simulink model "hexacopter"  (R2023b)
settings: Solver=ode3  StartTime=0.0  StopTime=inf  FixedStep=0.005  RelTol=1e-3
values from neighbouring files (symbols this model uses):
  A = [zeros(4),eye(4) ... (first row only)    [hexacopter_params.m]
  B = [0 0 0 0 ... (first row only)    [hexa.m]    (also in hexacopter_params.m = [zeros(4))
  body_params = [L,b,d,m,Ix,Iy,Iz,J_T]    [hexacopter_params.m]
  C = eye(8)    [hexacopter_params.m]
  g = 9.82    [hexacopter_params.m]
  K = place(A', C', desired_poles)'    [hexacopter_params.m]
  m = 2.5    [hexacopter_params.m]
  Simulation_params = [g,K_phi,K_theta,K_psi,K_x,K_y,K_z]    [hexacopter_params.m]
  T = [1, 1, 1, 1, 1, 1 ... (first row only)    [hexacopter_params.m]
  T_inv = pinv(T)    [hexacopter_params.m]
libraries: slpidlib x5, aerolibutil x2, vrlib x2
(part 1 of 2)
settings Model: Creator=alexe  LastModifiedBy=Therkelsen

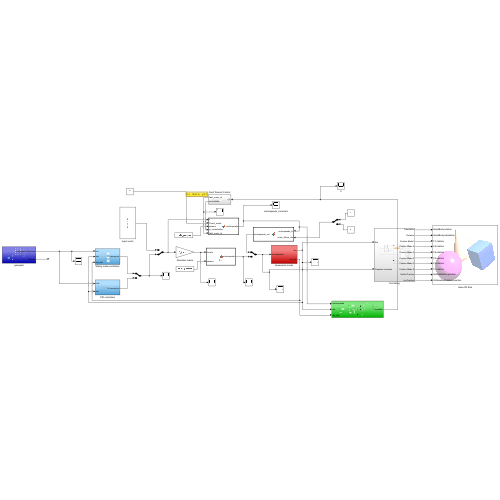
[thumbnail: Simulink's stored preview of the top-level diagram]
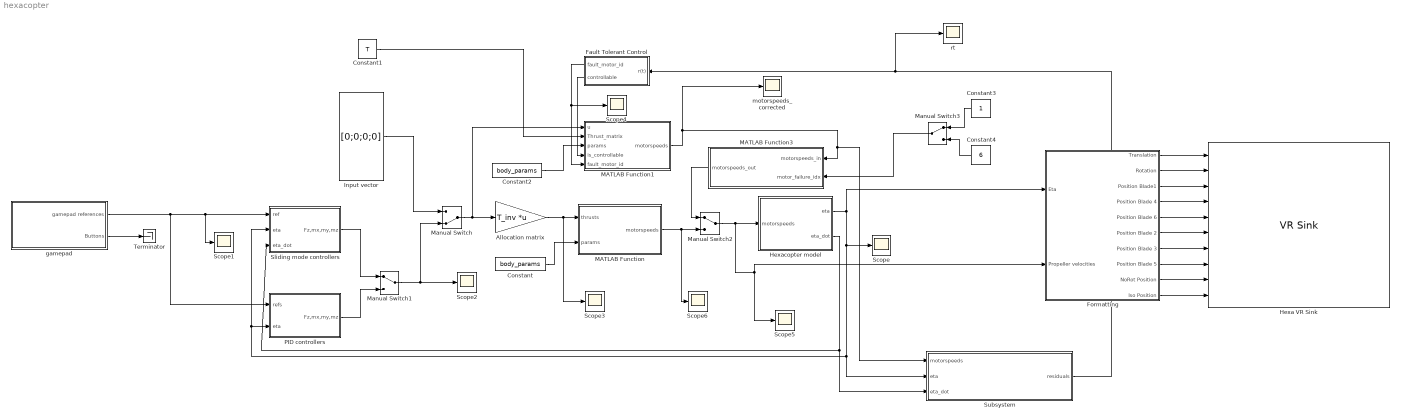
== system hexacopter ==
  Allocation matrix : Gain  Gain=T_inv  Multiplication=Matrix(K*u)
  Constant : Constant  Value=body_params
  Constant1 : Constant  Value=T
  Constant2 : Constant  Value=body_params
  Constant3 : Constant
  Constant4 : Constant  Value=6
  Fault Tolerant Control : Subsystem
  Formatting : Subsystem
  Hexa VR Sink : vrlib/VR Sink  InstantiateOnLoad=on  SampleTime=12*0.005  ViewEnable=on  RemoteChange=off  RemoteView=off  FieldsWritten=QuadBody.rotation.4.1.1.double#QuadBody.translation.3.1.1.double#F1.rotation.4.1.1.double#F4.rotation.4.1.1.double#F6.rotation.4.1.1.double#F2.rotation.4.1.1.double#F3.rotation.4.1.1.double#F5.rotation.4.1.1.double#IsoNoRotation.position.3.1.1.double#OnQuadNoRotation.position.3.1.1.double  WorldFileName=Hexacopter_VR.wrl  AutoView=on  VideoDimensions=[]  AllowVariableSize=off
  Hexacopter model : Subsystem
  Input vector : Constant  Value=[0;0;0;0]  VectorParams1D=off
  MATLAB Function : MATLAB Function  TreatAsAtomicUnit=on
  MATLAB Function1 : MATLAB Function  TreatAsAtomicUnit=on
  MATLAB Function3 : MATLAB Function  TreatAsAtomicUnit=on
  Manual Switch : ManualSwitch  CurrentSetting=0
  Manual Switch1 : ManualSwitch
  Manual Switch2 : ManualSwitch
  Manual Switch3 : ManualSwitch
  PID controllers : Subsystem
  Scope{,1..6} (7 alike) : Scope
  Sliding mode controllers : Subsystem
  Subsystem : Subsystem
  Terminator : Terminator
  gamepad : Subsystem
  motorspeeds_corrected : Scope
  rt : Scope
  wires:
  Allocation matrix/1 -> Scope3/1, MATLAB Function/1(thrusts)
  Manual Switch/1 -> MATLAB Function1/1(u), Allocation matrix/1
  Input vector/1 -> Manual Switch/1
  PID controllers/1(Fz,mx,my,mz) -> Manual Switch1/2
  Manual Switch1/1 -> Manual Switch/2, Scope2/1
  Sliding mode controllers/1(Fz,mx,my,mz) -> Manual Switch1/1
  Constant/1 -> MATLAB Function/2(params)
  Hexacopter model/2(eta_dot) -> Sliding mode controllers/3(eta_dot), Subsystem/3(eta_dot)
  MATLAB Function/1(motorspeeds) -> Scope6/1, Manual Switch2/2
  MATLAB Function1/1(motorspeeds) -> motorspeeds_corrected/1, Subsystem/1(motorspeeds), MATLAB Function3/1(motorspeeds_in)
  Constant2/1 -> MATLAB Function1/3(params)
  gamepad/1(gamepad references) -> PID controllers/1(refs), Scope1/1, Sliding mode controllers/1(ref)
  MATLAB Function3/1(motorspeeds_out) -> Manual Switch2/1
  Subsystem/1(residuals) -> rt/1, Fault Tolerant Control/1(r(t))
  Constant1/1 -> MATLAB Function1/2(Thrust_matrix)
  Fault Tolerant Control/2(controllable) -> MATLAB Function1/4(is_controllable)
  Constant4/1 -> Manual Switch3/2
  Manual Switch3/1 -> MATLAB Function3/2(motor_failure_idx)
  gamepad/2(Buttons) -> Terminator/1
  Fault Tolerant Control/1(fault_motor_id) -> Scope4/1, MATLAB Function1/5(fault_motor_id)
  Constant3/1 -> Manual Switch3/1
  Formatting/7(Position Blade 3) -> Hexa VR Sink/7
  Formatting/6(Position Blade 2) -> Hexa VR Sink/6
  Formatting/9(NoRot Position) -> Hexa VR Sink/9
  Formatting/10(Iso Position) -> Hexa VR Sink/10
  Formatting/3(Position Blade1) -> Hexa VR Sink/3
  Formatting/1(Translation) -> Hexa VR Sink/1
  Formatting/8(Position Blade 5) -> Hexa VR Sink/8
  Formatting/4(Position Blade 4) -> Hexa VR Sink/4
  Manual Switch2/1 -> Scope5/1, Formatting/2(Propeller velocities), Hexacopter model/1(motorspeeds)
  Formatting/5(Position Blade 6) -> Hexa VR Sink/5
  Hexacopter model/1(eta) -> Formatting/1(Eta), PID controllers/2(eta), Sliding mode controllers/2(eta), Subsystem/2(eta), Scope/1
  Formatting/2(Rotation) -> Hexa VR Sink/2

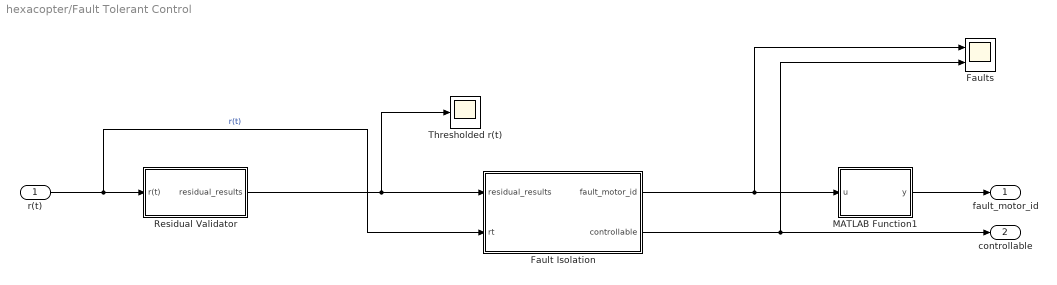
== system hexacopter/Fault Tolerant Control ==
  r(t) : Inport
  Fault Isolation : Subsystem
  Faults : Scope  NumInputPorts=2
  MATLAB Function1 : MATLAB Function  TreatAsAtomicUnit=on
  Residual Validator : Subsystem
  Thresholded r(t) : Scope
  fault_motor_id : Outport
  controllable : Outport  Port=2
  wires:
  Fault Isolation/1(fault_motor_id) -> MATLAB Function1/1(u), Faults/1
  Fault Isolation/2(controllable) -> Faults/2, controllable/1
  r(t)/1 -> Fault Isolation/2(rt), Residual Validator/1(r(t))  "r(t)"
  Residual Validator/1(residual_results) -> Fault Isolation/1(residual_results), Thresholded r(t)/1
  MATLAB Function1/1(y) -> fault_motor_id/1

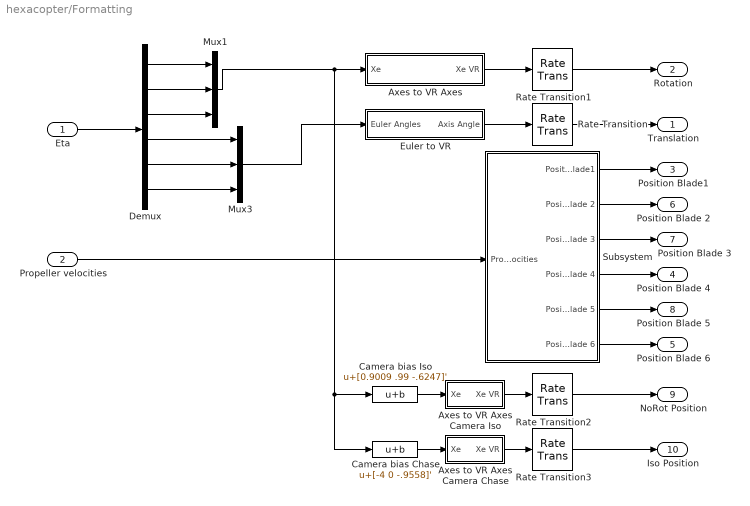
== system hexacopter/Formatting ==
  Eta : Inport
  Propeller velocities : Inport  Port=2
  Axes to VR Axes : Subsystem
  Axes to VR Axes Camera Chase : Subsystem
  Axes to VR Axes Camera Iso : Subsystem
  Camera bias Chase : Bias  Bias=[-4 0 -.9558]'  SaturateOnIntegerOverflow=off
  Camera bias Iso : Bias  Bias=[0.9009 .99 -.6247]'  SaturateOnIntegerOverflow=off
  Demux : Demux  Outputs=6
  Euler to VR : Subsystem
  Mux1 : Mux  Inputs=3
  Mux3 : Mux  Inputs=3
  Rate Transition{,1..3} (4 alike) : RateTransition
  Subsystem : Subsystem
  Translation : Outport
  Rotation : Outport  Port=2
  Position Blade1 : Outport  Port=3
  Position Blade 4 : Outport  Port=4
  Position Blade 6 : Outport  Port=5
  Position Blade 2 : Outport  Port=6
  Position Blade 3 : Outport  Port=7
  Position Blade 5 : Outport  Port=8
  NoRot Position : Outport  Port=9
  Iso Position : Outport  Port=10
  wires:
  Rate Transition2/1 -> NoRot Position/1
  Propeller velocities/1 -> Subsystem/1(Propeller velocities)
  Subsystem/3(Position Blade 3) -> Position Blade 3/1
  Subsystem/1(Position Blade1) -> Position Blade1/1
  Mux3/1 -> Euler to VR/1(Euler Angles)
  Camera bias Chase/1 -> Axes to VR Axes Camera Chase/1(Xe)
  Axes to VR Axes Camera Chase/1(Xe VR) -> Rate Transition3/1
  Subsystem/2(Position Blade 2) -> Position Blade 2/1
  Axes to VR Axes Camera Iso/1(Xe VR) -> Rate Transition2/1
  Euler to VR/1(Axis Angle) -> Rate Transition/1
  Axes to VR Axes/1(Xe VR) -> Rate Transition1/1
  Rate Transition1/1 -> Rotation/1
  Camera bias Iso/1 -> Axes to VR Axes Camera Iso/1(Xe)
  Mux1/1 -> Camera bias Chase/1, Camera bias Iso/1, Axes to VR Axes/1(Xe)
  Rate Transition3/1 -> Iso Position/1
  Rate Transition/1 -> Translation/1
  Subsystem/4(Position Blade 4) -> Position Blade 4/1
  Demux/2 -> Mux1/2
  Demux/5 -> Mux3/2
  Demux/3 -> Mux1/3
  Eta/1 -> Demux/1
  Demux/1 -> Mux1/1
  Demux/4 -> Mux3/1
  Demux/6 -> Mux3/3
  Subsystem/6(Position Blade 6) -> Position Blade 6/1
  Subsystem/5(Position Blade 5) -> Position Blade 5/1

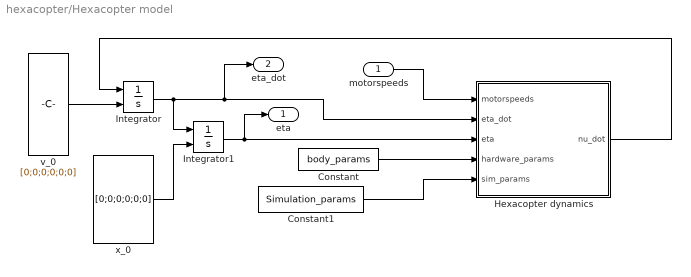
== system hexacopter/Hexacopter model ==
  motorspeeds : Inport
  Constant : Constant  Value=body_params
  Constant1 : Constant  Value=Simulation_params
  Hexacopter dynamics : MATLAB Function  TreatAsAtomicUnit=on
  Integrator : Integrator  InitialConditionSource=external
  Integrator1 : Integrator  InitialConditionSource=external
  v_0 : Constant  Value=[0;0;0;0;0;0]  VectorParams1D=off
  x_0 : Constant  Value=[0;0;0;0;0;0]  VectorParams1D=off
  eta : Outport
  eta_dot : Outport  Port=2
  wires:
  motorspeeds/1 -> Hexacopter dynamics/1(motorspeeds)
  Integrator/1 -> Integrator1/1, Hexacopter dynamics/2(eta_dot), eta_dot/1
  Integrator1/1 -> Hexacopter dynamics/3(eta), eta/1
  Hexacopter dynamics/1(nu_dot) -> Integrator/1
  v_0/1 -> Integrator/2
  Constant1/1 -> Hexacopter dynamics/5(sim_params)
  x_0/1 -> Integrator1/2
  Constant/1 -> Hexacopter dynamics/4(hardware_params)

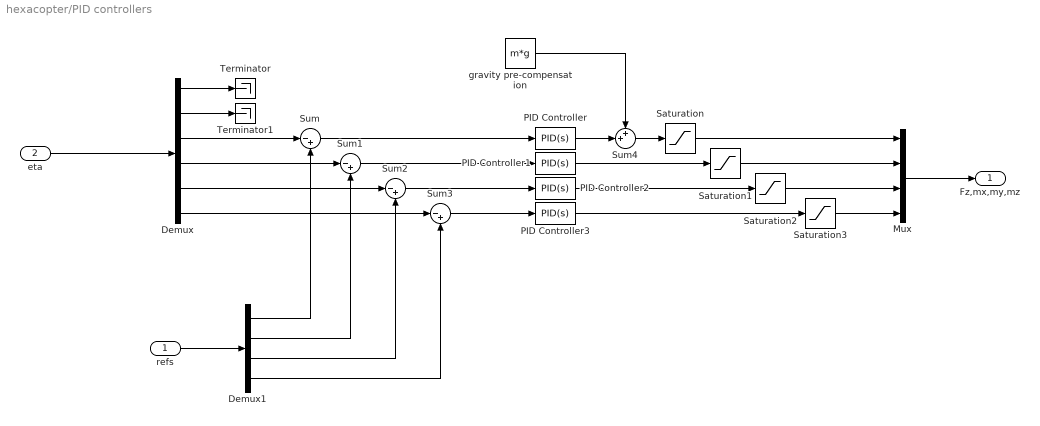
== system hexacopter/PID controllers ==
  refs : Inport
  eta : Inport  Port=2
  Demux : Demux  Outputs=6
  Demux1 : Demux
  Mux : Mux
  PID Controller : slpidlib/PID Controller  Controller=PID  Form=Parallel  TimeDomain=Continuous-time  UseExternalTs=off  SampleTime=-1  IntegratorMethod=Forward Euler  FilterMethod=Forward Euler  ControllerParametersSource=internal  P=3  I=1  UseKiTs=off  D=8  N=100  UseFilter=on  TunerSelectOption=Transfer Function Based (PID Tuner App)  InitialConditionSource=internal  InitialConditionForIntegrator=0  InitialConditionForFilter=0  DifferentiatorICPrevScaledInput=0  ExternalReset=none  TrackingMode=off  Kt=1  LimitOutput=off  SatLimitsSource=internal  UpperSaturationLimit=inf  LowerSaturationLimit=-inf  LinearizeAsGain=on  AntiWindupMode=none  Kb=1  LimitIntegrator=off  UpperIntegratorSaturationLimit=inf  LowerIntegratorSaturationLimit=-inf  POutMin=[]  POutMax=[]  IOutMin=[]  IOutMax=[]  DOutMin=[]  DOutMax=[]  NOutMin=[]  NOutMax=[]  SumOutMin=[]  SumOutMax=[]  SaturationOutMin=[]  SaturationOutMax=[]  PParamMin=[]  PParamMax=[]  IParamMin=[]  IParamMax=[]  DParamMin=[]  DParamMax=[]  NParamMin=[]  NParamMax=[]  KbParamMin=[]  KbParamMax=[]  KtParamMin=[]  KtParamMax=[]  KbOutMin=[]  KbOutMax=[]  KtOutMin=[]  KtOutMax=[]  IntegratorOutMin=[]  IntegratorOutMax=[]  FilterOutMin=[]  FilterOutMax=[]  SumI1OutMin=[]  SumI1OutMax=[]  SumI2OutMin=[]  SumI2OutMax=[]  SumI3OutMin=[]  SumI3OutMax=[]  SumI4OutMin=[]  SumI4OutMax=[]  SumDOutMin=[]  SumDOutMax=[]  DifferentiatorOutMin=[]  DifferentiatorOutMax=[]  FilterDiffOutCoefMin=[]  FilterDiffOutCoefMax=[]  ReciprocalOutMin=[]  ReciprocalOutMax=[]  SumDenOutMin=[]  SumDenOutMax=[]  SumNumOutMin=[]  SumNumOutMax=[]  DivideOutMin=[]  DivideOutMax=[]  UdiffTsProdOutMin=[]  UdiffTsProdOutMax=[]  NTsProdOutMin=[]  NTsProdOutMax=[]  UintegralTsProdOutMin=[]  UintegralTsProdOutMax=[]  UngainTsProdOutMin=[]  UngainTsProdOutMax=[]  ClampingZeroOutDataTypeStr=Inherit: Inherit via back propagation  ClampingZeroOutMin=[]  ClampingZeroOutMax=[]  FilterDenConstantOutDataTypeStr=Inherit: Inherit via back propagation  FilterDenConstantOutMin=[]  FilterDenConstantOutMax=[]  PCopyOutDataTypeStr=Inherit: Inherit via back propagation  PCopyOutMin=[]  PCopyOutMax=[]  NCopyOutDataTypeStr=Inherit: Inherit via back propagation  NCopyOutMin=[]  NCopyOutMax=[]  IntegratorContinuousStateAttributes=''  IntegratorStateMustResolveToSignalObject=off  IntegratorRTWStateStorageClass=Auto  FilterContinuousStateAttributes=''  FilterStateMustResolveToSignalObject=off  FilterRTWStateStorageClass=Auto  ParallelPVariant=InternalParameters  IdealPVariant=Disabled  IVariant=InternalParameters  DVariant=InternalParameters  IntegratorVariant=Continuous  SatVariant=Disabled  AWVariant=Passthrough  PCopyVariant=Disabled  TRVariant=Disabled  FdbkBlocksVariant=Forward  IdealPFdbkVariant=Disabled  SatFdbkVariant=Disabled  DerivativeFilterVariant=ContFilter  NVariant=InternalParameters  NCopyVariant=Disabled  FilterICVariant=InternalICsFilter  IntegratorICVariant=InternalICs  ExternalResetVariant=Disabled  TRSumVariant=Passthrough  SumFdbkVariant=Disabled  SumVariant=Sum_PID  TsampFilterVariant=InternalTs  TsampNgainVariant=Passthrough  TsampIntegralVariant=Disabled_SignalSpec  ExternalSaturationOutDataTypeStr=Inherit: Same as second input
  PID Controller1 : slpidlib/PID Controller  Controller=PID  Form=Parallel  TimeDomain=Continuous-time  UseExternalTs=off  SampleTime=-1  IntegratorMethod=Forward Euler  FilterMethod=Forward Euler  ControllerParametersSource=internal  P=1  I=0  UseKiTs=off  D=5  N=100  UseFilter=on  TunerSelectOption=Transfer Function Based (PID Tuner App)  InitialConditionSource=internal  InitialConditionForIntegrator=0  InitialConditionForFilter=0  DifferentiatorICPrevScaledInput=0  ExternalReset=none  TrackingMode=off  Kt=1  LimitOutput=off  SatLimitsSource=internal  UpperSaturationLimit=inf  LowerSaturationLimit=-inf  LinearizeAsGain=on  AntiWindupMode=none  Kb=1  LimitIntegrator=off  UpperIntegratorSaturationLimit=inf  LowerIntegratorSaturationLimit=-inf  POutMin=[]  POutMax=[]  IOutMin=[]  IOutMax=[]  DOutMin=[]  DOutMax=[]  NOutMin=[]  NOutMax=[]  SumOutMin=[]  SumOutMax=[]  SaturationOutMin=[]  SaturationOutMax=[]  PParamMin=[]  PParamMax=[]  IParamMin=[]  IParamMax=[]  DParamMin=[]  DParamMax=[]  NParamMin=[]  NParamMax=[]  KbParamMin=[]  KbParamMax=[]  KtParamMin=[]  KtParamMax=[]  KbOutMin=[]  KbOutMax=[]  KtOutMin=[]  KtOutMax=[]  IntegratorOutMin=[]  IntegratorOutMax=[]  FilterOutMin=[]  FilterOutMax=[]  SumI1OutMin=[]  SumI1OutMax=[]  SumI2OutMin=[]  SumI2OutMax=[]  SumI3OutMin=[]  SumI3OutMax=[]  SumI4OutMin=[]  SumI4OutMax=[]  SumDOutMin=[]  SumDOutMax=[]  DifferentiatorOutMin=[]  DifferentiatorOutMax=[]  FilterDiffOutCoefMin=[]  FilterDiffOutCoefMax=[]  ReciprocalOutMin=[]  ReciprocalOutMax=[]  SumDenOutMin=[]  SumDenOutMax=[]  SumNumOutMin=[]  SumNumOutMax=[]  DivideOutMin=[]  DivideOutMax=[]  UdiffTsProdOutMin=[]  UdiffTsProdOutMax=[]  NTsProdOutMin=[]  NTsProdOutMax=[]  UintegralTsProdOutMin=[]  UintegralTsProdOutMax=[]  UngainTsProdOutMin=[]  UngainTsProdOutMax=[]  ClampingZeroOutDataTypeStr=Inherit: Inherit via back propagation  ClampingZeroOutMin=[]  ClampingZeroOutMax=[]  FilterDenConstantOutDataTypeStr=Inherit: Inherit via back propagation  FilterDenConstantOutMin=[]  FilterDenConstantOutMax=[]  PCopyOutDataTypeStr=Inherit: Inherit via back propagation  PCopyOutMin=[]  PCopyOutMax=[]  NCopyOutDataTypeStr=Inherit: Inherit via back propagation  NCopyOutMin=[]  NCopyOutMax=[]  IntegratorContinuousStateAttributes=''  IntegratorStateMustResolveToSignalObject=off  IntegratorRTWStateStorageClass=Auto  FilterContinuousStateAttributes=''  FilterStateMustResolveToSignalObject=off  FilterRTWStateStorageClass=Auto  ParallelPVariant=InternalParameters  IdealPVariant=Disabled  IVariant=InternalParameters  DVariant=InternalParameters  IntegratorVariant=Continuous  SatVariant=Disabled  AWVariant=Passthrough  PCopyVariant=Disabled  TRVariant=Disabled  FdbkBlocksVariant=Forward  IdealPFdbkVariant=Disabled  SatFdbkVariant=Disabled  DerivativeFilterVariant=ContFilter  NVariant=InternalParameters  NCopyVariant=Disabled  FilterICVariant=InternalICsFilter  IntegratorICVariant=InternalICs  ExternalResetVariant=Disabled  TRSumVariant=Passthrough  SumFdbkVariant=Disabled  SumVariant=Sum_PID  TsampFilterVariant=InternalTs  TsampNgainVariant=Passthrough  TsampIntegralVariant=Disabled_SignalSpec  ExternalSaturationOutDataTypeStr=Inherit: Same as second input
  PID Controller2 : slpidlib/PID Controller  Controller=PID  Form=Parallel  TimeDomain=Continuous-time  UseExternalTs=off  SampleTime=-1  IntegratorMethod=Forward Euler  FilterMethod=Forward Euler  ControllerParametersSource=internal  P=1  I=0  UseKiTs=off  D=5  N=100  UseFilter=on  TunerSelectOption=Transfer Function Based (PID Tuner App)  InitialConditionSource=internal  InitialConditionForIntegrator=0  InitialConditionForFilter=0  DifferentiatorICPrevScaledInput=0  ExternalReset=none  TrackingMode=off  Kt=1  LimitOutput=off  SatLimitsSource=internal  UpperSaturationLimit=inf  LowerSaturationLimit=-inf  LinearizeAsGain=on  AntiWindupMode=none  Kb=1  LimitIntegrator=off  UpperIntegratorSaturationLimit=inf  LowerIntegratorSaturationLimit=-inf  POutMin=[]  POutMax=[]  IOutMin=[]  IOutMax=[]  DOutMin=[]  DOutMax=[]  NOutMin=[]  NOutMax=[]  SumOutMin=[]  SumOutMax=[]  SaturationOutMin=[]  SaturationOutMax=[]  PParamMin=[]  PParamMax=[]  IParamMin=[]  IParamMax=[]  DParamMin=[]  DParamMax=[]  NParamMin=[]  NParamMax=[]  KbParamMin=[]  KbParamMax=[]  KtParamMin=[]  KtParamMax=[]  KbOutMin=[]  KbOutMax=[]  KtOutMin=[]  KtOutMax=[]  IntegratorOutMin=[]  IntegratorOutMax=[]  FilterOutMin=[]  FilterOutMax=[]  SumI1OutMin=[]  SumI1OutMax=[]  SumI2OutMin=[]  SumI2OutMax=[]  SumI3OutMin=[]  SumI3OutMax=[]  SumI4OutMin=[]  SumI4OutMax=[]  SumDOutMin=[]  SumDOutMax=[]  DifferentiatorOutMin=[]  DifferentiatorOutMax=[]  FilterDiffOutCoefMin=[]  FilterDiffOutCoefMax=[]  ReciprocalOutMin=[]  ReciprocalOutMax=[]  SumDenOutMin=[]  SumDenOutMax=[]  SumNumOutMin=[]  SumNumOutMax=[]  DivideOutMin=[]  DivideOutMax=[]  UdiffTsProdOutMin=[]  UdiffTsProdOutMax=[]  NTsProdOutMin=[]  NTsProdOutMax=[]  UintegralTsProdOutMin=[]  UintegralTsProdOutMax=[]  UngainTsProdOutMin=[]  UngainTsProdOutMax=[]  ClampingZeroOutDataTypeStr=Inherit: Inherit via back propagation  ClampingZeroOutMin=[]  ClampingZeroOutMax=[]  FilterDenConstantOutDataTypeStr=Inherit: Inherit via back propagation  FilterDenConstantOutMin=[]  FilterDenConstantOutMax=[]  PCopyOutDataTypeStr=Inherit: Inherit via back propagation  PCopyOutMin=[]  PCopyOutMax=[]  NCopyOutDataTypeStr=Inherit: Inherit via back propagation  NCopyOutMin=[]  NCopyOutMax=[]  IntegratorContinuousStateAttributes=''  IntegratorStateMustResolveToSignalObject=off  IntegratorRTWStateStorageClass=Auto  FilterContinuousStateAttributes=''  FilterStateMustResolveToSignalObject=off  FilterRTWStateStorageClass=Auto  ParallelPVariant=InternalParameters  IdealPVariant=Disabled  IVariant=InternalParameters  DVariant=InternalParameters  IntegratorVariant=Continuous  SatVariant=Disabled  AWVariant=Passthrough  PCopyVariant=Disabled  TRVariant=Disabled  FdbkBlocksVariant=Forward  IdealPFdbkVariant=Disabled  SatFdbkVariant=Disabled  DerivativeFilterVariant=ContFilter  NVariant=InternalParameters  NCopyVariant=Disabled  FilterICVariant=InternalICsFilter  IntegratorICVariant=InternalICs  ExternalResetVariant=Disabled  TRSumVariant=Passthrough  SumFdbkVariant=Disabled  SumVariant=Sum_PID  TsampFilterVariant=InternalTs  TsampNgainVariant=Passthrough  TsampIntegralVariant=Disabled_SignalSpec  ExternalSaturationOutDataTypeStr=Inherit: Same as second input
  PID Controller3 : slpidlib/PID Controller  Controller=PID  Form=Parallel  TimeDomain=Continuous-time  UseExternalTs=off  SampleTime=-1  IntegratorMethod=Forward Euler  FilterMethod=Forward Euler  ControllerParametersSource=internal  P=1  I=0  UseKiTs=off  D=3  N=100  UseFilter=on  TunerSelectOption=Transfer Function Based (PID Tuner App)  InitialConditionSource=internal  InitialConditionForIntegrator=0  InitialConditionForFilter=0  DifferentiatorICPrevScaledInput=0  ExternalReset=none  TrackingMode=off  Kt=1  LimitOutput=off  SatLimitsSource=internal  UpperSaturationLimit=inf  LowerSaturationLimit=-inf  LinearizeAsGain=on  AntiWindupMode=none  Kb=1  LimitIntegrator=off  UpperIntegratorSaturationLimit=inf  LowerIntegratorSaturationLimit=-inf  POutMin=[]  POutMax=[]  IOutMin=[]  IOutMax=[]  DOutMin=[]  DOutMax=[]  NOutMin=[]  NOutMax=[]  SumOutMin=[]  SumOutMax=[]  SaturationOutMin=[]  SaturationOutMax=[]  PParamMin=[]  PParamMax=[]  IParamMin=[]  IParamMax=[]  DParamMin=[]  DParamMax=[]  NParamMin=[]  NParamMax=[]  KbParamMin=[]  KbParamMax=[]  KtParamMin=[]  KtParamMax=[]  KbOutMin=[]  KbOutMax=[]  KtOutMin=[]  KtOutMax=[]  IntegratorOutMin=[]  IntegratorOutMax=[]  FilterOutMin=[]  FilterOutMax=[]  SumI1OutMin=[]  SumI1OutMax=[]  SumI2OutMin=[]  SumI2OutMax=[]  SumI3OutMin=[]  SumI3OutMax=[]  SumI4OutMin=[]  SumI4OutMax=[]  SumDOutMin=[]  SumDOutMax=[]  DifferentiatorOutMin=[]  DifferentiatorOutMax=[]  FilterDiffOutCoefMin=[]  FilterDiffOutCoefMax=[]  ReciprocalOutMin=[]  ReciprocalOutMax=[]  SumDenOutMin=[]  SumDenOutMax=[]  SumNumOutMin=[]  SumNumOutMax=[]  DivideOutMin=[]  DivideOutMax=[]  UdiffTsProdOutMin=[]  UdiffTsProdOutMax=[]  NTsProdOutMin=[]  NTsProdOutMax=[]  UintegralTsProdOutMin=[]  UintegralTsProdOutMax=[]  UngainTsProdOutMin=[]  UngainTsProdOutMax=[]  ClampingZeroOutDataTypeStr=Inherit: Inherit via back propagation  ClampingZeroOutMin=[]  ClampingZeroOutMax=[]  FilterDenConstantOutDataTypeStr=Inherit: Inherit via back propagation  FilterDenConstantOutMin=[]  FilterDenConstantOutMax=[]  PCopyOutDataTypeStr=Inherit: Inherit via back propagation  PCopyOutMin=[]  PCopyOutMax=[]  NCopyOutDataTypeStr=Inherit: Inherit via back propagation  NCopyOutMin=[]  NCopyOutMax=[]  IntegratorContinuousStateAttributes=''  IntegratorStateMustResolveToSignalObject=off  IntegratorRTWStateStorageClass=Auto  FilterContinuousStateAttributes=''  FilterStateMustResolveToSignalObject=off  FilterRTWStateStorageClass=Auto  ParallelPVariant=InternalParameters  IdealPVariant=Disabled  IVariant=InternalParameters  DVariant=InternalParameters  IntegratorVariant=Continuous  SatVariant=Disabled  AWVariant=Passthrough  PCopyVariant=Disabled  TRVariant=Disabled  FdbkBlocksVariant=Forward  IdealPFdbkVariant=Disabled  SatFdbkVariant=Disabled  DerivativeFilterVariant=ContFilter  NVariant=InternalParameters  NCopyVariant=Disabled  FilterICVariant=InternalICsFilter  IntegratorICVariant=InternalICs  ExternalResetVariant=Disabled  TRSumVariant=Passthrough  SumFdbkVariant=Disabled  SumVariant=Sum_PID  TsampFilterVariant=InternalTs  TsampNgainVariant=Passthrough  TsampIntegralVariant=Disabled_SignalSpec  ExternalSaturationOutDataTypeStr=Inherit: Same as second input
  Saturation : Saturate  UpperLimit=100  LowerLimit=-100
  Saturation1 : Saturate  UpperLimit=5  LowerLimit=-5
  Saturation2 : Saturate  UpperLimit=5  LowerLimit=-5
  Saturation3 : Saturate  UpperLimit=5  LowerLimit=-5
  Sum{,1..3} (4 alike) : Sum  Inputs=|-+
  Sum4 : Sum  Inputs=++|
  Terminator : Terminator
  Terminator1 : Terminator
  gravity pre-compensation : Constant  Value=m*g
  Fz,mx,my,mz : Outport
  wires:
  eta/1 -> Demux/1
  refs/1 -> Demux1/1
  Demux/1 -> Terminator/1
  Demux/2 -> Terminator1/1
  Demux/3 -> Sum/1
  Demux1/1 -> Sum/2
  Demux/4 -> Sum1/1
  Demux1/2 -> Sum1/2
  Demux/5 -> Sum2/1
  Demux1/3 -> Sum2/2
  Demux/6 -> Sum3/1
  Demux1/4 -> Sum3/2
  Sum/1 -> PID Controller/1
  Sum1/1 -> PID Controller1/1
  Sum2/1 -> PID Controller2/1
  Sum3/1 -> PID Controller3/1
  PID Controller3/1 -> Saturation3/1
  PID Controller2/1 -> Saturation2/1
  PID Controller1/1 -> Saturation1/1
  Mux/1 -> Fz,mx,my,mz/1
  Sum4/1 -> Saturation/1
  PID Controller/1 -> Sum4/2
  gravity pre-compensation/1 -> Sum4/1
  Saturation/1 -> Mux/1
  Saturation1/1 -> Mux/2
  Saturation2/1 -> Mux/3
  Saturation3/1 -> Mux/4

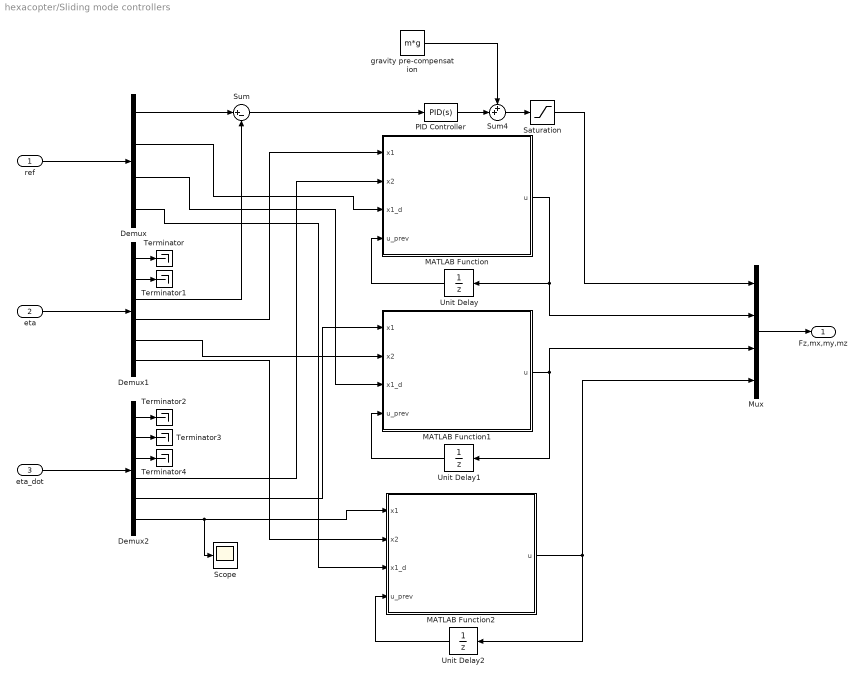
== system hexacopter/Sliding mode controllers ==
  ref : Inport
  eta : Inport  Port=2
  eta_dot : Inport  Port=3
  Demux : Demux
  Demux1 : Demux  Outputs=6
  Demux2 : Demux  Outputs=6
  MATLAB Function : MATLAB Function  TreatAsAtomicUnit=on
  MATLAB Function1 : MATLAB Function  TreatAsAtomicUnit=on
  MATLAB Function2 : MATLAB Function  TreatAsAtomicUnit=on
  Mux : Mux
  PID Controller : slpidlib/PID Controller  Controller=PID  Form=Parallel  TimeDomain=Continuous-time  UseExternalTs=off  SampleTime=-1  IntegratorMethod=Forward Euler  FilterMethod=Forward Euler  ControllerParametersSource=internal  P=3  I=1  UseKiTs=off  D=8  N=100  UseFilter=on  TunerSelectOption=Transfer Function Based (PID Tuner App)  InitialConditionSource=internal  InitialConditionForIntegrator=0  InitialConditionForFilter=0  DifferentiatorICPrevScaledInput=0  ExternalReset=none  TrackingMode=off  Kt=1  LimitOutput=off  SatLimitsSource=internal  UpperSaturationLimit=inf  LowerSaturationLimit=-inf  LinearizeAsGain=on  AntiWindupMode=none  Kb=1  LimitIntegrator=off  UpperIntegratorSaturationLimit=inf  LowerIntegratorSaturationLimit=-inf  POutMin=[]  POutMax=[]  IOutMin=[]  IOutMax=[]  DOutMin=[]  DOutMax=[]  NOutMin=[]  NOutMax=[]  SumOutMin=[]  SumOutMax=[]  SaturationOutMin=[]  SaturationOutMax=[]  PParamMin=[]  PParamMax=[]  IParamMin=[]  IParamMax=[]  DParamMin=[]  DParamMax=[]  NParamMin=[]  NParamMax=[]  KbParamMin=[]  KbParamMax=[]  KtParamMin=[]  KtParamMax=[]  KbOutMin=[]  KbOutMax=[]  KtOutMin=[]  KtOutMax=[]  IntegratorOutMin=[]  IntegratorOutMax=[]  FilterOutMin=[]  FilterOutMax=[]  SumI1OutMin=[]  SumI1OutMax=[]  SumI2OutMin=[]  SumI2OutMax=[]  SumI3OutMin=[]  SumI3OutMax=[]  SumI4OutMin=[]  SumI4OutMax=[]  SumDOutMin=[]  SumDOutMax=[]  DifferentiatorOutMin=[]  DifferentiatorOutMax=[]  FilterDiffOutCoefMin=[]  FilterDiffOutCoefMax=[]  ReciprocalOutMin=[]  ReciprocalOutMax=[]  SumDenOutMin=[]  SumDenOutMax=[]  SumNumOutMin=[]  SumNumOutMax=[]  DivideOutMin=[]  DivideOutMax=[]  UdiffTsProdOutMin=[]  UdiffTsProdOutMax=[]  NTsProdOutMin=[]  NTsProdOutMax=[]  UintegralTsProdOutMin=[]  UintegralTsProdOutMax=[]  UngainTsProdOutMin=[]  UngainTsProdOutMax=[]  ClampingZeroOutDataTypeStr=Inherit: Inherit via back propagation  ClampingZeroOutMin=[]  ClampingZeroOutMax=[]  FilterDenConstantOutDataTypeStr=Inherit: Inherit via back propagation  FilterDenConstantOutMin=[]  FilterDenConstantOutMax=[]  PCopyOutDataTypeStr=Inherit: Inherit via back propagation  PCopyOutMin=[]  PCopyOutMax=[]  NCopyOutDataTypeStr=Inherit: Inherit via back propagation  NCopyOutMin=[]  NCopyOutMax=[]  IntegratorContinuousStateAttributes=''  IntegratorStateMustResolveToSignalObject=off  IntegratorRTWStateStorageClass=Auto  FilterContinuousStateAttributes=''  FilterStateMustResolveToSignalObject=off  FilterRTWStateStorageClass=Auto  ParallelPVariant=InternalParameters  IdealPVariant=Disabled  IVariant=InternalParameters  DVariant=InternalParameters  IntegratorVariant=Continuous  SatVariant=Disabled  AWVariant=Passthrough  PCopyVariant=Disabled  TRVariant=Disabled  FdbkBlocksVariant=Forward  IdealPFdbkVariant=Disabled  SatFdbkVariant=Disabled  DerivativeFilterVariant=ContFilter  NVariant=InternalParameters  NCopyVariant=Disabled  FilterICVariant=InternalICsFilter  IntegratorICVariant=InternalICs  ExternalResetVariant=Disabled  TRSumVariant=Passthrough  SumFdbkVariant=Disabled  SumVariant=Sum_PID  TsampFilterVariant=InternalTs  TsampNgainVariant=Passthrough  TsampIntegralVariant=Disabled_SignalSpec  ExternalSaturationOutDataTypeStr=Inherit: Same as second input
  Saturation : Saturate  UpperLimit=100  LowerLimit=-100
  Scope : Scope
  Sum : Sum  Inputs=|+-
  Sum4 : Sum  Inputs=++|
  Terminator{,1..4} (5 alike) : Terminator
  Unit Delay : UnitDelay  SampleTime=-1  HasFrameUpgradeWarning=on
  Unit Delay1 : UnitDelay  SampleTime=-1  HasFrameUpgradeWarning=on
  Unit Delay2 : UnitDelay  SampleTime=-1  HasFrameUpgradeWarning=on
  gravity pre-compensation : Constant  Value=m*g
  Fz,mx,my,mz : Outport
  wires:
  ref/1 -> Demux/1
  Mux/1 -> Fz,mx,my,mz/1
  eta/1 -> Demux1/1
  eta_dot/1 -> Demux2/1
  Demux1/1 -> Terminator/1
  Demux1/2 -> Terminator1/1
  Demux2/1 -> Terminator2/1
  Demux2/2 -> Terminator3/1
  Demux1/4 -> MATLAB Function/1(x1)
  Demux2/4 -> MATLAB Function/2(x2)
  Demux/2 -> MATLAB Function/3(x1_d)
  MATLAB Function/1(u) -> Mux/2, Unit Delay/1
  Unit Delay/1 -> MATLAB Function/4(u_prev)
  MATLAB Function1/1(u) -> Unit Delay1/1, Mux/3
  Unit Delay1/1 -> MATLAB Function1/4(u_prev)
  Demux2/5 -> MATLAB Function1/1(x1)
  Demux1/5 -> MATLAB Function1/2(x2)
  Demux/3 -> MATLAB Function1/3(x1_d)
  MATLAB Function2/1(u) -> Unit Delay2/1, Mux/4
  Unit Delay2/1 -> MATLAB Function2/4(u_prev)
  Demux2/6 -> Scope/1, MATLAB Function2/1(x1)
  Demux1/6 -> MATLAB Function2/2(x2)
  Demux/4 -> MATLAB Function2/3(x1_d)
  Sum/1 -> PID Controller/1
  gravity pre-compensation/1 -> Sum4/1
  PID Controller/1 -> Sum4/2
  Sum4/1 -> Saturation/1
  Demux/1 -> Sum/1
  Demux1/3 -> Sum/2
  Saturation/1 -> Mux/1
  Demux2/3 -> Terminator4/1

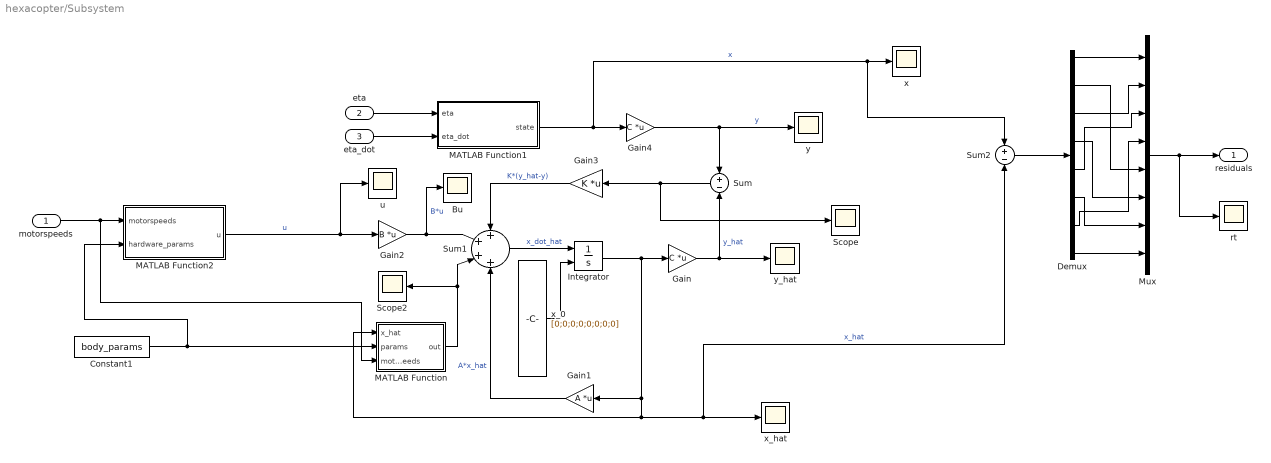
== system hexacopter/Subsystem ==
  motorspeeds : Inport
  eta : Inport  Port=2
  eta_dot : Inport  Port=3
  Bu : Scope
  Constant1 : Constant  Value=body_params
  Demux : Demux  Outputs=8
  Gain : Gain  Gain=C  Multiplication=Matrix(K*u)
  Gain1 : Gain  Gain=A  Multiplication=Matrix(K*u)
  Gain2 : Gain  Gain=B  Multiplication=Matrix(K*u)
  Gain3 : Gain  Gain=K  Multiplication=Matrix(K*u)
  Gain4 : Gain  Gain=C  Multiplication=Matrix(K*u)
  Integrator : Integrator  InitialConditionSource=external
  MATLAB Function : MATLAB Function  TreatAsAtomicUnit=on
  MATLAB Function1 : MATLAB Function  TreatAsAtomicUnit=on
  MATLAB Function2 : MATLAB Function  TreatAsAtomicUnit=on
  Mux : Mux  Inputs=8
  Scope : Scope
  Scope2 : Scope
  Sum : Sum  Inputs=+|-
  Sum1 : Sum  Inputs=+|+|+|+
  Sum2 : Sum  Inputs=+|-
  rt : Scope
  u : Scope
  x : Scope
  x_0 : Constant  Value=[0;0;0;0;0;0;0;0]  VectorParams1D=off
  x_hat : Scope
  y : Scope
  y_hat : Scope
  residuals : Outport
  wires:
  MATLAB Function1/1(state) -> Sum2/1, x/1, Gain4/1  "x"
  Gain/1 -> y_hat/1, Sum/2  "y_hat"
  x_0/1 -> Integrator/2
  Sum1/1 -> Integrator/1  "x_dot_hat"
  Sum/1 -> Scope/1, Gain3/1
  Integrator/1 -> Sum2/2, x_hat/1, MATLAB Function/1(x_hat), Gain1/1, Gain/1  "x_hat"
  Gain2/1 -> Bu/1, Sum1/2  "B*u"
  Constant1/1 -> MATLAB Function2/2(hardware_params), MATLAB Function/2(params)
  motorspeeds/1 -> MATLAB Function/3(motorspeeds), MATLAB Function2/1(motorspeeds)
  eta_dot/1 -> MATLAB Function1/2(eta_dot)
  eta/1 -> MATLAB Function1/1(eta)
  Gain3/1 -> Sum1/1  "K*(y_hat-y)"
  Gain4/1 -> y/1, Sum/1  "y"
  Gain1/1 -> Sum1/4  "A*x_hat"
  MATLAB Function/1(out) -> Scope2/1, Sum1/3
  MATLAB Function2/1(u) -> u/1, Gain2/1  "u"
  Sum2/1 -> Demux/1
  Demux/1 -> Mux/1
  Demux/2 -> Mux/5
  Demux/3 -> Mux/2
  Demux/4 -> Mux/6
  Demux/5 -> Mux/3
  Demux/6 -> Mux/7
  Demux/7 -> Mux/4
  Demux/8 -> Mux/8
  Mux/1 -> rt/1, residuals/1

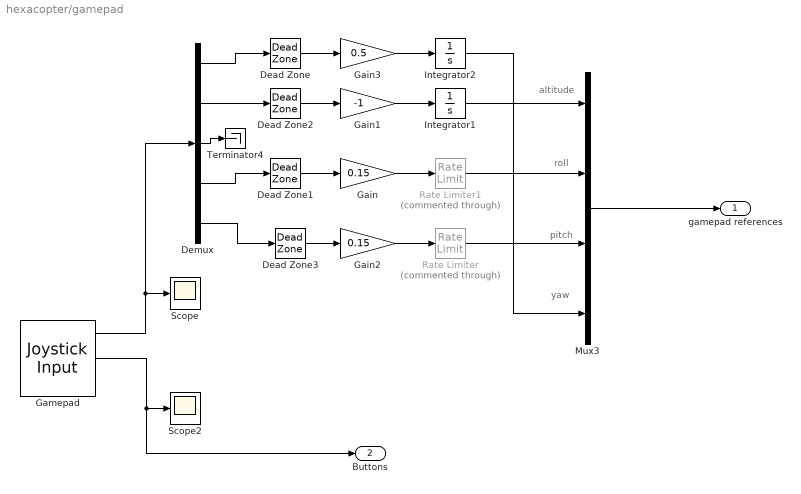
== system hexacopter/gamepad ==
  note: roll
  note: altitude
  note: pitch
  note: yaw
  Dead Zone{,1..3} (4 alike) : DeadZone  LowerValue=-0.2  UpperValue=0.2
  Demux : Demux  Outputs=5
  Gain : Gain  Gain=0.15
  Gain1 : Gain  Gain=-1
  Gain2 : Gain  Gain=0.15
  Gain3 : Gain  Gain=0.5
  Gamepad : vrlib/Joystick Input  joyid=1  adjustports=on  forcefeed=off
  Integrator1 : Integrator
  Integrator2 : Integrator
  Mux3 : Mux
  Rate Limiter : RateLimiter  Commented=through  RisingSlewLimit=0.2  FallingSlewLimit=-0.2  SampleTimeMode=inherited
  Rate Limiter1 : RateLimiter  Commented=through  RisingSlewLimit=0.2  FallingSlewLimit=-0.2  SampleTimeMode=inherited
  Scope : Scope
  Scope2 : Scope
  Terminator4 : Terminator
  gamepad references : Outport
  Buttons : Outport  Port=2
  wires:
  Gamepad/2 -> Buttons/1, Scope2/1
  Gain2/1 -> Rate Limiter/1
  Integrator1/1 -> Mux3/1
  Demux/3 -> Terminator4/1
  Rate Limiter1/1 -> Mux3/2
  Gain3/1 -> Integrator2/1
  Dead Zone/1 -> Gain3/1
  Demux/5 -> Dead Zone3/1
  Mux3/1 -> gamepad references/1
  Gain/1 -> Rate Limiter1/1
  Gain1/1 -> Integrator1/1
  Demux/2 -> Dead Zone2/1
  Demux/1 -> Dead Zone/1
  Rate Limiter/1 -> Mux3/3
  Integrator2/1 -> Mux3/4
  Dead Zone3/1 -> Gain2/1
  Demux/4 -> Dead Zone1/1
  Dead Zone1/1 -> Gain/1
  Dead Zone2/1 -> Gain1/1
  Gamepad/1 -> Demux/1, Scope/1

== system hexacopter/Fault Tolerant Control/Fault Isolation ==
  residual_results : Inport
  rt : Inport  Port=2
  MATLAB Function : MATLAB Function  TreatAsAtomicUnit=on
  fault_motor_id : Outport
  controllable : Outport  Port=2
  wires:
  MATLAB Function/1(fault_motor_id) -> fault_motor_id/1
  MATLAB Function/2(controllable) -> controllable/1
  residual_results/1 -> MATLAB Function/1(r)
  rt/1 -> MATLAB Function/2(rt)

== system hexacopter/Fault Tolerant Control/Residual Validator ==
  r(t) : Inport
  Hi : Constant  Value=0.5
  Mi : Constant  Value=-0.5
  Single Motor Residual Validator : MATLAB Function  TreatAsAtomicUnit=on
  residual_results : Outport
  wires:
  r(t)/1 -> Single Motor Residual Validator/1(r)
  Hi/1 -> Single Motor Residual Validator/3(Hi)
  Mi/1 -> Single Motor Residual Validator/2(Mi)
  Single Motor Residual Validator/1(residual_results) -> residual_results/1  "4x1 vector (r5 - r8) -1 -> ri < Mi 0 -> Mi <= ri <= Hi 1 -> ri > Hi"

== system hexacopter/Formatting/Axes to VR Axes ==
  Xe : Inport
  Demux : Demux  Outputs=3
      settings: DisplayOption=none
  Mux : Mux  Inputs=3
  rad-->deg1 : Gain  SaturateOnIntegerOverflow=on  OutDataTypeStr=Inherit: Same as input  ParamDataTypeStr=Inherit: Same as input
  Xe VR : Outport  VectorParamsAs1DForOutWhenUnconnected=off
  wires:
  Xe/1 -> Demux/1
  Demux/1 -> Mux/1
  Demux/3 -> rad-->deg1/1
  Mux/1 -> Xe VR/1
  rad-->deg1/1 -> Mux/2
  Demux/2 -> Mux/3

== system hexacopter/Formatting/Axes to VR Axes Camera Chase ==
  Xe : Inport
  Demux : Demux  Outputs=3
      settings: DisplayOption=none
  Mux : Mux  Inputs=3
  rad-->deg1 : Gain  Gain=-1  SaturateOnIntegerOverflow=on  OutDataTypeStr=Inherit: Same as input  ParamDataTypeStr=Inherit: Same as input
  Xe VR : Outport  VectorParamsAs1DForOutWhenUnconnected=off
  wires:
  Xe/1 -> Demux/1
  Demux/1 -> Mux/1
  Demux/3 -> rad-->deg1/1
  Mux/1 -> Xe VR/1
  rad-->deg1/1 -> Mux/2
  Demux/2 -> Mux/3

== system hexacopter/Formatting/Axes to VR Axes Camera Iso ==
  Xe : Inport
  Demux : Demux  Outputs=3
      settings: DisplayOption=none
  Mux : Mux  Inputs=3
  rad-->deg1 : Gain  Gain=-1  SaturateOnIntegerOverflow=on  OutDataTypeStr=Inherit: Same as input  ParamDataTypeStr=Inherit: Same as input
  Xe VR : Outport  VectorParamsAs1DForOutWhenUnconnected=off
  wires:
  Demux/2 -> Mux/3
  rad-->deg1/1 -> Mux/2
  Mux/1 -> Xe VR/1
  Demux/3 -> rad-->deg1/1
  Demux/1 -> Mux/1
  Xe/1 -> Demux/1

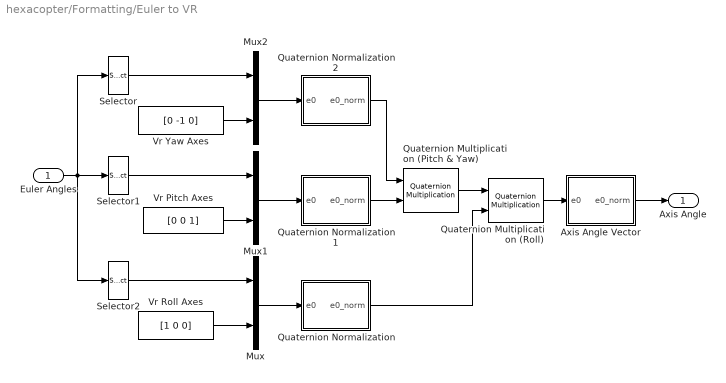
== system hexacopter/Formatting/Euler to VR ==
  Euler Angles : Inport
  Axis Angle Vector : Subsystem
  Mux : Mux  Inputs=2
  Mux1 : Mux  Inputs=2
  Mux2 : Mux  Inputs=2
  Quaternion Multiplication (Pitch & Yaw) : aerolibutil/Quaternion Multiplication
  Quaternion Multiplication (Roll) : aerolibutil/Quaternion Multiplication
  Quaternion Normalization : Subsystem
  Quaternion Normalization1 : Subsystem
  Quaternion Normalization2 : Subsystem
  Selector : Selector  InputPortWidth=3  IndexOptions=Index vector (dialog)  Indices=[3]  OutputSizes=1
  Selector1 : Selector  InputPortWidth=3  IndexOptions=Index vector (dialog)  Indices=[2]  OutputSizes=1
  Selector2 : Selector  InputPortWidth=3  IndexOptions=Index vector (dialog)  Indices=[1]  OutputSizes=1
  Vr Pitch Axes : Constant  Value=[0 0 1]
  Vr Roll Axes : Constant  Value=[1 0 0]
  Vr Yaw Axes : Constant  Value=[0 -1 0]
  Axis Angle : Outport  VectorParamsAs1DForOutWhenUnconnected=off
  wires:
  Quaternion Multiplication (Roll)/1 -> Axis Angle Vector/1(e0)
  Axis Angle Vector/1(e0_norm) -> Axis Angle/1
  Quaternion Normalization/1(e0_norm) -> Quaternion Multiplication (Roll)/2
  Quaternion Normalization2/1(e0_norm) -> Quaternion Multiplication (Pitch & Yaw)/1
  Quaternion Normalization1/1(e0_norm) -> Quaternion Multiplication (Pitch & Yaw)/2
  Mux2/1 -> Quaternion Normalization2/1(e0)
  Mux1/1 -> Quaternion Normalization1/1(e0)
  Mux/1 -> Quaternion Normalization/1(e0)
  Selector/1 -> Mux2/1
  Vr Yaw Axes/1 -> Mux2/2
  Selector1/1 -> Mux1/1
  Vr Pitch Axes/1 -> Mux1/2
  Selector2/1 -> Mux/1
  Vr Roll Axes/1 -> Mux/2
  Euler Angles/1 -> Selector2/1, Selector1/1, Selector/1
  Quaternion Multiplication (Pitch & Yaw)/1 -> Quaternion Multiplication (Roll)/1

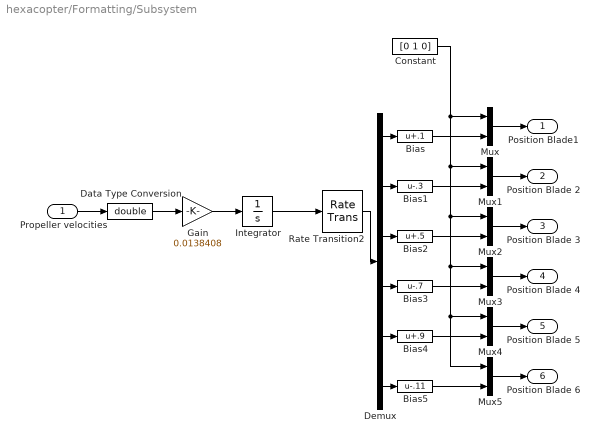
== system hexacopter/Formatting/Subsystem ==
  Propeller velocities : Inport
  Bias : Bias  Bias=.1  SaturateOnIntegerOverflow=off
  Bias1 : Bias  Bias=-.3  SaturateOnIntegerOverflow=off
  Bias2 : Bias  Bias=.5  SaturateOnIntegerOverflow=off
  Bias3 : Bias  Bias=-.7  SaturateOnIntegerOverflow=off
  Bias4 : Bias  Bias=.9  SaturateOnIntegerOverflow=off
  Bias5 : Bias  Bias=-.11  SaturateOnIntegerOverflow=off
  Constant : Constant  Value=[0 1 0]
  Data Type Conversion : DataTypeConversion  OutDataTypeStr=double  SaturateOnIntegerOverflow=off  RndMeth=Floor
  Demux : Demux  Outputs=6
  Gain : Gain  Gain=0.0138408
  Integrator : Integrator  InitialCondition=[.1 ; .2 ;-.3 ;-.4;-.5;-.6]  WrapState=on  WrappedStateUpperValue=2*pi  WrappedStateLowerValue=-2*pi
  Mux{,1..5} (6 alike) : Mux  Inputs=2
  Rate Transition2 : RateTransition
  Position Blade1 : Outport  VectorParamsAs1DForOutWhenUnconnected=off
  Position Blade 2 : Outport  Port=2  VectorParamsAs1DForOutWhenUnconnected=off
  Position Blade 3 : Outport  Port=3  VectorParamsAs1DForOutWhenUnconnected=off
  Position Blade 4 : Outport  Port=4  VectorParamsAs1DForOutWhenUnconnected=off
  Position Blade 5 : Outport  Port=5  VectorParamsAs1DForOutWhenUnconnected=off
  Position Blade 6 : Outport  Port=6  VectorParamsAs1DForOutWhenUnconnected=off
  wires:
  Bias3/1 -> Mux3/2
  Mux3/1 -> Position Blade 4/1
  Bias1/1 -> Mux1/2
  Bias2/1 -> Mux2/2
  Demux/2 -> Bias1/1
  Mux1/1 -> Position Blade 2/1
  Mux2/1 -> Position Blade 3/1
  Integrator/1 -> Rate Transition2/1
  Mux/1 -> Position Blade1/1
  Demux/3 -> Bias2/1
  Bias/1 -> Mux/2
  Propeller velocities/1 -> Data Type Conversion/1
  Demux/4 -> Bias3/1
  Rate Transition2/1 -> Demux/1
  Demux/1 -> Bias/1
  Data Type Conversion/1 -> Gain/1
  Gain/1 -> Integrator/1
  Demux/6 -> Bias5/1
  Demux/5 -> Bias4/1
  Mux5/1 -> Position Blade 6/1
  Bias4/1 -> Mux4/2
  Mux4/1 -> Position Blade 5/1
  Bias5/1 -> Mux5/2
  Constant/1 -> Mux5/1, Mux4/1, Mux3/1, Mux2/1, Mux1/1, Mux/1

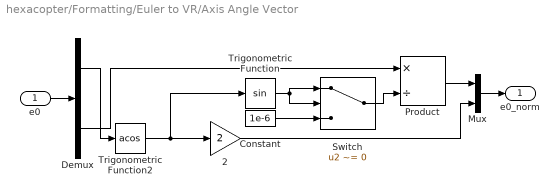
== system hexacopter/Formatting/Euler to VR/Axis Angle Vector ==
  e0 : Inport
  2 : Gain  Gain=2  SaturateOnIntegerOverflow=on  OutDataTypeStr=Inherit: Same as input  ParamDataTypeStr=Inherit: Same as input
  Constant : Constant  Value=1e-6
  Demux : Demux  Outputs=[1 3 ]
      settings: DisplayOption=none
  Mux : Mux  Inputs=2
  Product : Product  Inputs=*/  InputSameDT=on  SaturateOnIntegerOverflow=on  OutDataTypeStr=Inherit: Same as first input
  Switch : Switch  Criteria=u2 ~= 0  SaturateOnIntegerOverflow=off  InputSameDT=off
  Trigonometric Function : Trigonometry
  Trigonometric Function2 : Trigonometry  Operator=acos
  e0_norm : Outport  VectorParamsAs1DForOutWhenUnconnected=off
  wires:
  Demux/1 -> Trigonometric Function2/1
  Demux/2 -> Product/1
  Mux/1 -> e0_norm/1
  Product/1 -> Mux/1
  2/1 -> Mux/2
  Trigonometric Function/1 -> Switch/1, Switch/2
  Trigonometric Function2/1 -> Trigonometric Function/1, 2/1
  e0/1 -> Demux/1
  Constant/1 -> Switch/3
  Switch/1 -> Product/2

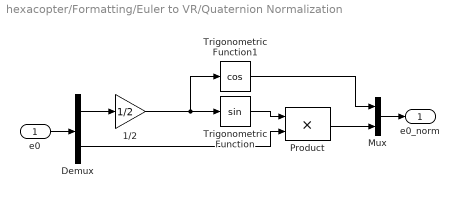
== system hexacopter/Formatting/Euler to VR/Quaternion Normalization ==
  e0 : Inport
  1/2 : Gain  Gain=1/2  SaturateOnIntegerOverflow=on  OutDataTypeStr=Inherit: Same as input  ParamDataTypeStr=Inherit: Same as input
  Demux : Demux  Outputs=[1 3]
      settings: DisplayOption=none
  Mux : Mux  Inputs=2
  Product : Product  InputSameDT=on  SaturateOnIntegerOverflow=on  OutDataTypeStr=Inherit: Same as first input
  Trigonometric Function : Trigonometry
  Trigonometric Function1 : Trigonometry  Operator=cos
  e0_norm : Outport  VectorParamsAs1DForOutWhenUnconnected=off
  wires:
  Trigonometric Function1/1 -> Mux/1
  Demux/2 -> Product/2
  Demux/1 -> 1/2/1
  Mux/1 -> e0_norm/1
  Product/1 -> Mux/2
  Trigonometric Function/1 -> Product/1
  1/2/1 -> Trigonometric Function1/1, Trigonometric Function/1
  e0/1 -> Demux/1

== system hexacopter/Formatting/Euler to VR/Quaternion Normalization1 ==
  e0 : Inport
  1/2 : Gain  Gain=1/2  SaturateOnIntegerOverflow=on  OutDataTypeStr=Inherit: Same as input  ParamDataTypeStr=Inherit: Same as input
  Demux : Demux  Outputs=[1 3]
      settings: DisplayOption=none
  Mux : Mux  Inputs=2
  Product : Product  InputSameDT=on  SaturateOnIntegerOverflow=on  OutDataTypeStr=Inherit: Same as first input
  Trigonometric Function : Trigonometry
  Trigonometric Function1 : Trigonometry  Operator=cos
  e0_norm : Outport  VectorParamsAs1DForOutWhenUnconnected=off
  wires:
  e0/1 -> Demux/1
  1/2/1 -> Trigonometric Function/1, Trigonometric Function1/1
  Trigonometric Function/1 -> Product/1
  Product/1 -> Mux/2
  Mux/1 -> e0_norm/1
  Demux/1 -> 1/2/1
  Demux/2 -> Product/2
  Trigonometric Function1/1 -> Mux/1

== system hexacopter/Formatting/Euler to VR/Quaternion Normalization2 ==
  e0 : Inport
  1/2 : Gain  Gain=1/2  SaturateOnIntegerOverflow=on  OutDataTypeStr=Inherit: Same as input  ParamDataTypeStr=Inherit: Same as input
  Demux : Demux  Outputs=[1 3]
      settings: DisplayOption=none
  Mux : Mux  Inputs=2
  Product : Product  InputSameDT=on  SaturateOnIntegerOverflow=on  OutDataTypeStr=Inherit: Same as first input
  Trigonometric Function : Trigonometry
  Trigonometric Function1 : Trigonometry  Operator=cos
  e0_norm : Outport  VectorParamsAs1DForOutWhenUnconnected=off
  wires:
  Trigonometric Function1/1 -> Mux/1
  Demux/2 -> Product/2
  Demux/1 -> 1/2/1
  Mux/1 -> e0_norm/1
  Product/1 -> Mux/2
  Trigonometric Function/1 -> Product/1
  1/2/1 -> Trigonometric Function1/1, Trigonometric Function/1
  e0/1 -> Demux/1

== matlab function hexacopter/Fault Tolerant Control/Residual Validator/Single Motor Residual Validator ==
  data: r input; residual_results output; Mi input; Hi input
function residual_results = validate_residuals(r, Mi, Hi)
    %r = r(5:8);
    residual_results = zeros(size(r));
    residual_results(r < Mi) = -1;
    residual_results(r > Hi) = 1;
end

== matlab function hexacopter/Sliding mode controllers/MATLAB Function2 ==
  settings: updateMethod=DISCRETE
  data: x1 input; u output; x2 input; x1_d input; u_prev input
function u = SMC_Attitude(x1, x2, x1_d, u_prev)
% SMC with constant reference (assumes dx1_d = 0, ddx1_d = 0)

Iz = 0.01187; % moment of inertia z [kg*m^2]
h = 1/Iz;

f = 0;
% k      = 5;
% Gamma  = 25;
% delta  = 2;

k      = 1;
Gamma  = 20;
delta  = 0.1;

% k      = 0;
% Gamma  = 20*h;
% delta  = 0;

persistent z_i
if isempty(z_i)
    z_i = 0;
end
e = (x1 - x1_d);
de = x2;  % dx1_d = 0
s = de + k * e;
d_hat = z_i + delta * x2;
dz = -delta * z_i - delta * (delta * x2 + f + h * u_prev);
z_i = z_i + dz * 0.005;  % 200 Hz
if abs(s) <= 1
    sat_s = s;
else
    sat_s = sign(s);
end
u = (-f - d_hat - k * de - Gamma * sat_s) / h;

== matlab function hexacopter/Fault Tolerant Control/MATLAB Function1 ==
  settings: updateMethod=DISCRETE
  data: u input; y output
function y = holdFirstChange(u)
%#codegen

persistent initial_value;
persistent has_changed;
persistent latched_value;

if isempty(initial_value)
    initial_value = u;
    has_changed = false;
    latched_value = u;
end

if ~has_changed && any(u ~= initial_value)
    latched_value = u;
    has_changed = true;
end

if has_changed
    y = latched_value;
else
    y = u;
end

== matlab function hexacopter/Subsystem/MATLAB Function1 ==
  data: eta input; state output; eta_dot input
function state = fcn(eta,eta_dot)

state = [eta(4);
         eta_dot(4);
         eta(5);
         eta_dot(5);
         eta(6);
         eta_dot(6);
         eta(3);
         eta_dot(3)];

== matlab function hexacopter/MATLAB Function ==
  data: thrusts input; motorspeeds output; params input
function motorspeeds = fcn(thrusts,params)

b = params(2); % Thrust coefficient [N/m^2]

% motorspeeds = sqrt(max(0,thrusts)/b);

nonneg_speeds = max(thrusts,0);
nonneg_indexes = find(thrusts<0);

for i=1:length(nonneg_indexes)
    idx = nonneg_indexes(i);
    if mod(idx,2)==0
        nonneg_speeds(idx-1) = nonneg_speeds(idx-1)+abs(thrusts(idx));
    else
        nonneg_speeds(idx+1) = nonneg_speeds(idx+1)+abs(thrusts(idx));
    end
end

motorspeeds = sqrt(nonneg_speeds/b);

motorspeeds = sqrt(max(0,thrusts)/b);

== matlab function hexacopter/Hexacopter model/Hexacopter dynamics ==
  data: nu_dot output; motorspeeds input; eta_dot input; eta input; hardware_params input; sim_params input
function nu_dot = fcn(motorspeeds,eta_dot,eta,hardware_params,sim_params)

L = hardware_params(1);
b = hardware_params(2);
d = hardware_params(3);
m = hardware_params(4);
Ix = hardware_params(5);
Iy = hardware_params(6);
Iz = hardware_params(7);
J_T = hardware_params(8);

F1 = b*motorspeeds(1)^2;
F2 = b*motorspeeds(2)^2;
F3 = b*motorspeeds(3)^2;
F4 = b*motorspeeds(4)^2;
F5 = b*motorspeeds(5)^2;
F6 = b*motorspeeds(6)^2;

tau1 = d*motorspeeds(1)^2;
tau2 = d*motorspeeds(2)^2;
tau3 = d*motorspeeds(3)^2;
tau4 = d*motorspeeds(4)^2;
tau5 = d*motorspeeds(5)^2;
tau6 = d*motorspeeds(6)^2;

U1 = F1+F2+F3+F4+F5+F6;
U2 = (F2-F1+(F3+F6-F4-F5)/2)*L;
U3 = (F3+F5-F4-F6)*L*sqrt(3)/2;
U4 = tau2+tau5+tau6-tau1-tau3-tau4;

g = sim_params(1);
K_phi = sim_params(2);
K_theta = sim_params(3);
K_psi = sim_params(4);
K_x = sim_params(5);
K_y = sim_params(6);
K_z = sim_params(7);

phi = eta(4);
theta = eta(5);
psi = eta(6);

x_dot = eta_dot(1);
y_dot = eta_dot(2); 
z_dot = eta_dot(3);
phi_dot = eta_dot(4);
theta_dot = eta_dot(5);
psi_dot = eta_dot(6);


Omega = motorspeeds(3)+motorspeeds(4)-motorspeeds(1)-motorspeeds(2);
% max_omega = 1;  % Maximum yaw rate (in rad/s)
% Omega = max(min(Omega, max_omega), -max_omega);  % Saturate Omega

nu_dot = zeros(6,1);
nu_dot(1) = (-U1*(cos(phi)*sin(theta)*cos(psi)+sin(phi)*sin(psi))-K_x*x_dot)/m;
nu_dot(2) = (-U1*(cos(phi)*sin(theta)*sin(psi)-sin(phi)*sin(psi))-K_y*y_dot)/m;
nu_dot(3) = -g+(U1*(cos(phi)*cos(theta))-K_z*z_dot)/m;
nu_dot(4) = (U2+(Iy-Iz)*theta_dot*psi_dot-J_T*theta_dot*Omega-K_phi*phi_dot)/Ix;
nu_dot(5) = (U3+(Iz-Ix)*phi_dot*psi_dot-J_T*phi_dot*Omega-K_theta*theta_dot)/Iy;
nu_dot(6) = (U4+(Ix-Iy)*phi_dot*theta_dot-K_psi*psi_dot)/Iz;

== matlab function hexacopter/Subsystem/MATLAB Function2 ==
  data: motorspeeds input; u output; hardware_params input
function u = fcn(motorspeeds,hardware_params)

L = hardware_params(1);
b = hardware_params(2);
d = hardware_params(3);

F1 = b*motorspeeds(1)^2;
F2 = b*motorspeeds(2)^2;
F3 = b*motorspeeds(3)^2;
F4 = b*motorspeeds(4)^2;
F5 = b*motorspeeds(5)^2;
F6 = b*motorspeeds(6)^2;

tau1 = d*motorspeeds(1)^2;
tau2 = d*motorspeeds(2)^2;
tau3 = d*motorspeeds(3)^2;
tau4 = d*motorspeeds(4)^2;
tau5 = d*motorspeeds(5)^2;
tau6 = d*motorspeeds(6)^2;

U1 = F1+F2+F3+F4+F5+F6;
U2 = (F2-F1+(F3+F6-F4-F5)/2)*L;
U3 = (F3+F5-F4-F6)*L*sqrt(3)/2;
U4 = tau2+tau5+tau6-tau1-tau3-tau4;

u = [U2;U3;U4;U1];

== matlab function hexacopter/Subsystem/MATLAB Function ==
  data: x_hat input; params input; motorspeeds input; out output
function out = h(x_hat,params,motorspeeds)

Ix = params(5);
Iy = params(6);
Iz = params(7);
J_T = params(8);

g = 9.82;

phi_dot = x_hat(2);
theta_dot = x_hat(4);
psi_dot = x_hat(6);

Omega = motorspeeds(3)+motorspeeds(4)-motorspeeds(1)-motorspeeds(2);
% max_omega = 1;  % Maximum yaw rate (in rad/s)
% Omega = max(min(Omega, max_omega), -max_omega);  % Saturate Omega

out = [zeros(4,1);
       (theta_dot*psi_dot*(Iy-Iz)-J_T*theta_dot*Omega)/Ix;
       (phi_dot*psi_dot*(Iz-Ix)-J_T*phi_dot*Omega)/Iy;
       phi_dot*theta_dot*(Ix-Iy)/Iz;
       -g];

% out = zeros(8,1);

== matlab function hexacopter/MATLAB Function1 ==
  data: u input; motorspeeds output; Thrust_matrix input; params input; is_controllable input; fault_motor_id input
function motorspeeds = fcn(u, Thrust_matrix, params, is_controllable, fault_motor_id)

motor_coeff_b = params(2); % Thrust coefficient [N/m^2]
A = Thrust_matrix;
b = u;

fault_motor_id = 0;
if fault_motor_id <= 0 % CASE: Nothing wrong
    lambda = 0.1;
    A_aug = [A; sqrt(lambda) * eye(6)];
    b_aug = [b; zeros(6, 1)];
    thrusts = lsqnonneg(A_aug, b_aug);
    motorspeeds = sqrt(thrusts/motor_coeff_b);
    return
end

if fault_motor_id > 0
    % MAGI, men virker
    cols = true(1, size(A,2));
    cols(fault_motor_id) = false;
    A_reduced = A(:, cols);
    % End of magic
    
    lambda = 0.005;
    A_aug = [A_reduced; sqrt(lambda) * eye(5)];
    b_aug = [b; zeros(5, 1)];
    thrusts_reduced = lsqnonneg(A_aug, b_aug);

    %thrusts_reduced = lsqnonneg(A_reduced, b);

    thrusts_full = zeros(6,1);
    idx = 1;
    for i = 1:6
        if i == fault_motor_id
            thrusts_full(i) = 0;
        else
            thrusts_full(i) = thrusts_reduced(idx);
            idx = idx + 1;
        end
    end
    motorspeeds = sqrt(thrusts_full/motor_coeff_b);
    return
end

motorspeeds = zeros(6,1);

== matlab function hexacopter/Sliding mode controllers/MATLAB Function ==
  settings: updateMethod=DISCRETE
  data: x1 input; u output; x2 input; x1_d input; u_prev input
function u = SMC_Attitude(x1, x2, x1_d, u_prev)

Ix = 100*0.00915; % moment of inertia x [kg*m^2]
h = 1/Ix;

f = 0;
% k      = 6;
% Gamma  = 12;
% delta  = 3;

k      = 1;
Gamma  = 20;
delta  = 0.1;

% k      = 0;
% Gamma  = 20*h;
% delta  = 0;

persistent z_i
if isempty(z_i)
    z_i = 0;
end
e = x1 - x1_d;
de = x2;  % dx1_d = 0
s = de + k * e;
d_hat = z_i + delta * x2;
dz = -delta * z_i - delta * (delta * x2 + f + h * u_prev);
z_i = z_i + dz * 0.005;  % 200 Hz
if abs(s) <= 1
    sat_s = s;
else
    sat_s = sign(s);
end
u = (-f - d_hat - k * de - Gamma * sat_s) / h;

== matlab function hexacopter/MATLAB Function3 ==
  data: motorspeeds_in input; motorspeeds_out output; motor_failure_idx input
function motorspeeds_out = fcn(motorspeeds_in, motor_failure_idx)
    
motorspeeds_out = motorspeeds_in;
if(motor_failure_idx > 0)
    motorspeeds_out(motor_failure_idx) = 0;
end

== matlab function hexacopter/Fault Tolerant Control/Fault Isolation/MATLAB Function ==
  settings: updateMethod=DISCRETE
  data: r input; fault_motor_id output; controllable output; rt input
function [fault_motor_id, controllable] = fault_lookup(r,rt)
% r: 4x1 vector with values in {-1,0,1} for residuals 5..8

fault_patterns8d = [
  %r1   r2   r3   r4   r5   r6   r7   r8
  -1    0    0    1   -1    0    0    0;   % f1 CORRECT
   1    0   -1    1    0    0    0    0;   % f2 mixup with f6
  -1    0    1    1   -1    0    1    0;%-1;   % f3 CORRECT
  -1    0    0    1   -1    0    1    0;   % f4 CORRECT
   1    0   -1    1    1    0    1    0;   % f5 CORRECT
   1    0   -1    1    1    0    0    0;   % f6 mixup with f2
];

r_7d = [r(1:4);r(6:8)];
fault_patterns7d = [fault_patterns8d(:,1:4),fault_patterns8d(:,6:8)];

norm_threshold = 3.7;

% Define fault patterns as rows in a matrix (faults x 4 residuals)
% fault_patterns = [
%    %r5  %r6  %r7  %r8
%     1    0    1   -1;   % f1
%    -1    0   -1   -1;   % f2
%    -1   -1    1   -1;   % f3
%     1    1    1   -1;   % f4
%     1   -1   -1   -1;   % f5
%    -1    1   -1   -1;   % f6
% ];


controllability = [1; 1; 0; 1; 0; 1];  % 1 = Yes, 0 = No

% Initialize outputs
fault_motor_id = 0;         % No fault by default
controllable = false;

if norm(rt) > norm_threshold
for i = 1:size(fault_patterns8d,1)
    if isequal(r(:)', fault_patterns8d(i,:))
        fault_motor_id = i;
        controllable = logical(controllability(i));
        break;
    end
end
if all(r == 0)
    fault_motor_id = 0;
    controllable = true;
elseif fault_motor_id == 0
    fault_motor_id = -1;
    controllable = false;
end
end
end
